simulink model "control_STMD_Ideal_Entrega_Final"  (R2021b)
settings: Solver=ode4  StartTime=0.0  StopTime=tend  FixedStep=ts  RelTol=1e-3  EnableMultiTasking=on
values from neighbouring files (symbols this model uses):
  ct = 2*mt*(2*pi*ft)*dampt    [script_control_STMD_Ideal_Entrega_Final.m]
  Kmax = 1*ct    [script_control_STMD_Ideal_Entrega_Final.m]
  Kmin = ct/2    [script_control_STMD_Ideal_Entrega_Final.m]
  kt = ((2*pi*ft)^2)*mt    [script_control_STMD_Ideal_Entrega_Final.m]
  mt = mu*m1    (= 60)    [script_control_STMD_Ideal_Entrega_Final.m]
  tend = 15    [script_control_STMD_Ideal_Entrega_Final.m]
  ts = 1/fs    (= 0.000666666666667)    [script_control_STMD_Ideal_Entrega_Final.m]
  u_active = 200    [script_control_STMD_Ideal_Entrega_Final.m]
undefined symbols (not defined in the file or in its folder): D_Gs, N_Gs
libraries: simulink x1
settings Model: Creator=user  LastModifiedBy=luismiguelmartinezgomez
settings SolverCC: AlgebraicLoopSolver=TrustRegion
settings DataIOCC: LimitDataPoints=on  SaveFormat=Array  SignalLoggingSaveFormat=ModelDataLogs  ReturnWorkspaceOutputs=off  SignalLoggingName=sigsOut
settings OptimizationCC: InitFltsAndDblsToZero=on  LifeSpan=inf
settings DebuggingCC: SaveWithParameterizedLinksMsg=none  UnderspecifiedInitializationDetection=Classic  MergeDetectMultiDrivingBlocksExec=none  SignalResolutionControl=TryResolveAllWithWarning  MultiTaskDSMMsg=warning  MultiTaskCondExecSysMsg=none  FcnCallInpInsideContextMsg=warning  SFUnexpectedBacktrackingDiag=warning  SFNoUnconditionalDefaultTransitionDiag=warning  SFMachineParentedDataDiag=warning  ArithmeticOperatorsInVariantConditions=warning
settings HardwareCC: ProdBitPerPointer=32  ProdBitPerSizeT=32  ProdBitPerPtrDiffT=32  ProdLargestAtomicFloat=None  ProdIntDivRoundTo=Undefined  ProdEndianess=Unspecified  ProdWordSize=32  ProdHWDeviceType=32-bit Generic  TargetBitPerLong=64  TargetBitPerPointer=64  TargetBitPerSizeT=64  TargetBitPerPtrDiffT=64  TargetLongLongMode=on  TargetIntDivRoundTo=Zero  TargetEndianess=LittleEndian  TargetWordSize=64  TargetHWDeviceType=MATLAB Host  ProdEqTarget=off
settings ModelReferenceCC: PropagateSignalLabelsOutOfModel=off
settings SFSimCC: SimUseLocalCustomCode=off  CustomCodeUndefinedFunction=UseInterfaceOnly
settings RTWCC: RTWUseLocalCustomCode=off
settings CodeAppCC: StateflowObjectComments=on
settings GRTTargetCC: TargetFcnLib=ansi_tfl_tmw.mat  TargetLangStandard=C89/C90 (ANSI)  CombineOutputUpdateFcns=off  GRTInterface=on
settings ConfigComp: CovMetricSettings=dw  CovSaveCumulativeToWorkspaceVar=on  CovSaveSingleToWorkspaceVar=on  CovExternalEMLEnable=off  CovSFcnEnable=off

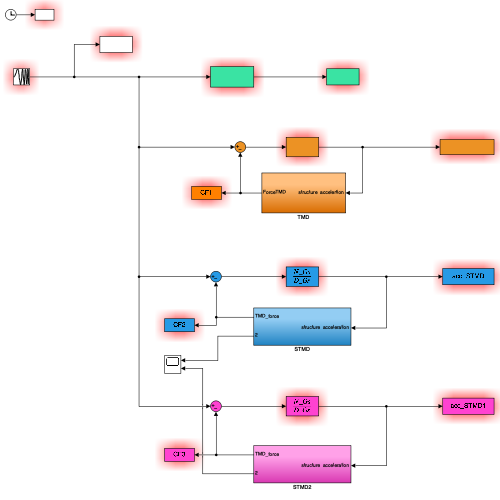
[thumbnail: Simulink's stored preview of the top-level diagram]
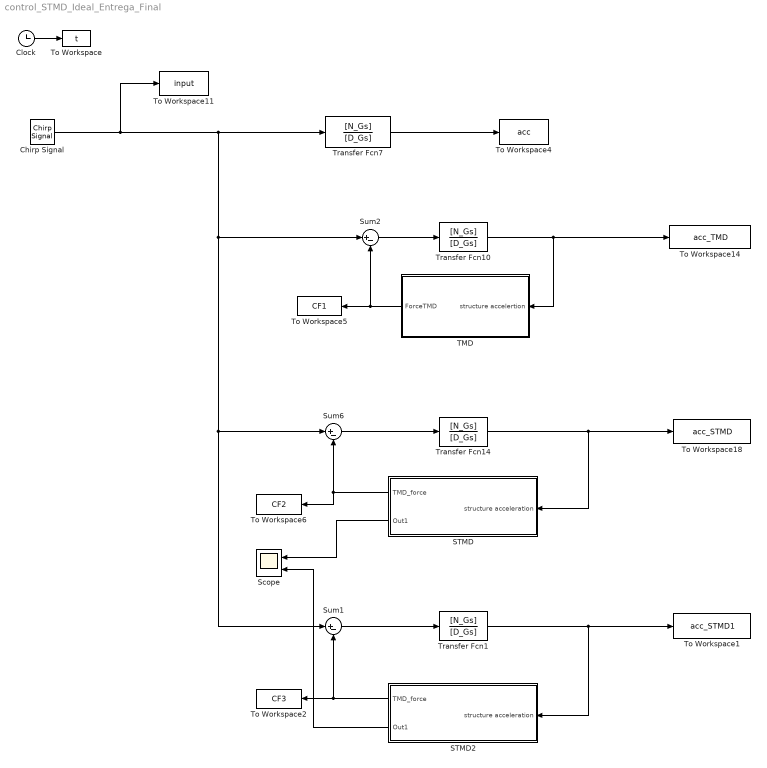
== system control_STMD_Ideal_Entrega_Final ==
  Chirp Signal : simulink/Sources/Chirp Signal  f1=fmin  T=tend  f2=fmax
  Clock : Clock
  STMD : Subsystem
  STMD2 : Subsystem
  Scope : Scope  NumInputPorts=2
  Sum1 : Sum  Inputs=|+-
  Sum2 : Sum  Inputs=|+-
  Sum6 : Sum  Inputs=|+-
  TMD : Subsystem
  To Workspace : ToWorkspace  VariableName=t  SampleTime=ts
  To Workspace1 : ToWorkspace  VariableName=acc_STMD1  SampleTime=ts
  To Workspace11 : ToWorkspace  VariableName=input  SampleTime=ts
  To Workspace14 : ToWorkspace  VariableName=acc_TMD  SampleTime=ts
  To Workspace18 : ToWorkspace  VariableName=acc_STMD  SampleTime=ts
  To Workspace2 : ToWorkspace  VariableName=CF3  SampleTime=ts
  To Workspace4 : ToWorkspace  VariableName=acc  SampleTime=ts
  To Workspace5 : ToWorkspace  VariableName=CF1  SampleTime=ts
  To Workspace6 : ToWorkspace  VariableName=CF2  SampleTime=ts
  Transfer Fcn{1,7,10,14} (4 alike) : TransferFcn  Numerator=[N_Gs]  Denominator=[D_Gs]
  wires:
  Clock/1 -> To Workspace/1
  Sum2/1 -> Transfer Fcn10/1
  TMD/1(ForceTMD) -> Sum2/2, To Workspace5/1
  Transfer Fcn7/1 -> To Workspace4/1
  Transfer Fcn10/1 -> TMD/1(structure accelertion), To Workspace14/1
  Sum6/1 -> Transfer Fcn14/1
  Transfer Fcn14/1 -> STMD/1(structure acceleration), To Workspace18/1
  STMD/1(TMD_force) -> To Workspace6/1, Sum6/2
  Chirp Signal/1 -> Sum2/1, Sum1/1, Sum6/1, Transfer Fcn7/1, To Workspace11/1
  STMD2/1(TMD_force) -> Sum1/2, To Workspace2/1
  Transfer Fcn1/1 -> STMD2/1(structure acceleration), To Workspace1/1
  Sum1/1 -> Transfer Fcn1/1
  STMD/2(Out1) -> Scope/1
  STMD2/2(Out1) -> Scope/2

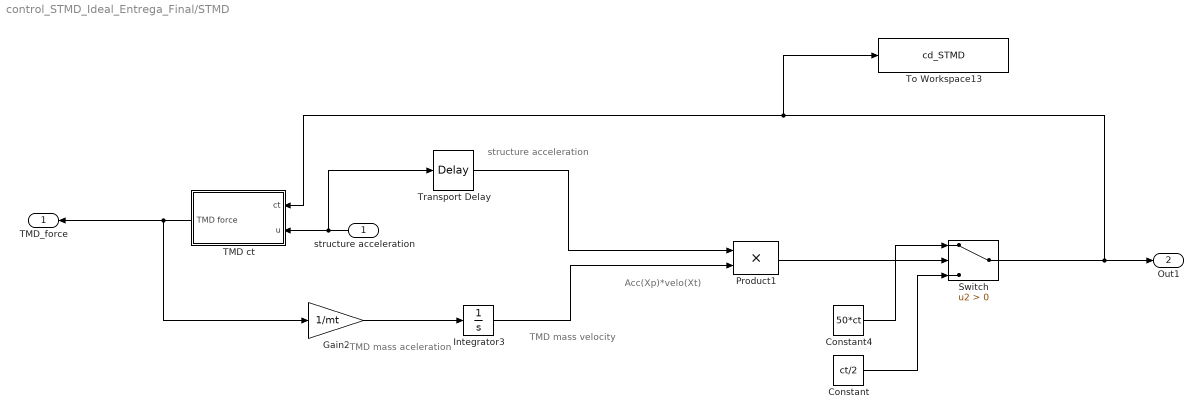
== system control_STMD_Ideal_Entrega_Final/STMD ==
  note: structure acceleration
  note: TMD mass
      | aceleration
  note: Acc(Xp)*velo(Xt)
  note: TMD mass
      | velocity
  structure acceleration : Inport
  Constant : Constant  Value=ct/2
  Constant4 : Constant  Value=50*ct
  Gain2 : Gain  Gain=1/mt
  Integrator3 : Integrator
  Product1 : Product  OutDataTypeStr=double  SaturateOnIntegerOverflow=on
  Switch : Switch  Criteria=u2 > Threshold
  TMD ct : Subsystem
  To Workspace13 : ToWorkspace  VariableName=cd_STMD  SampleTime=ts
  Transport Delay : TransportDelay  DelayTime=ts
  TMD_force : Outport  VectorParamsAs1DForOutWhenUnconnected=off
  Out1 : Outport  Port=2
  wires:
  TMD ct/1(TMD force) -> Gain2/1, TMD_force/1
  Integrator3/1 -> Product1/2
  Switch/1 -> Out1/1, To Workspace13/1, TMD ct/1(ct)
  structure acceleration/1 -> Transport Delay/1, TMD ct/2(u)
  Transport Delay/1 -> Product1/1
  Gain2/1 -> Integrator3/1
  Product1/1 -> Switch/2
  Constant4/1 -> Switch/1
  Constant/1 -> Switch/3

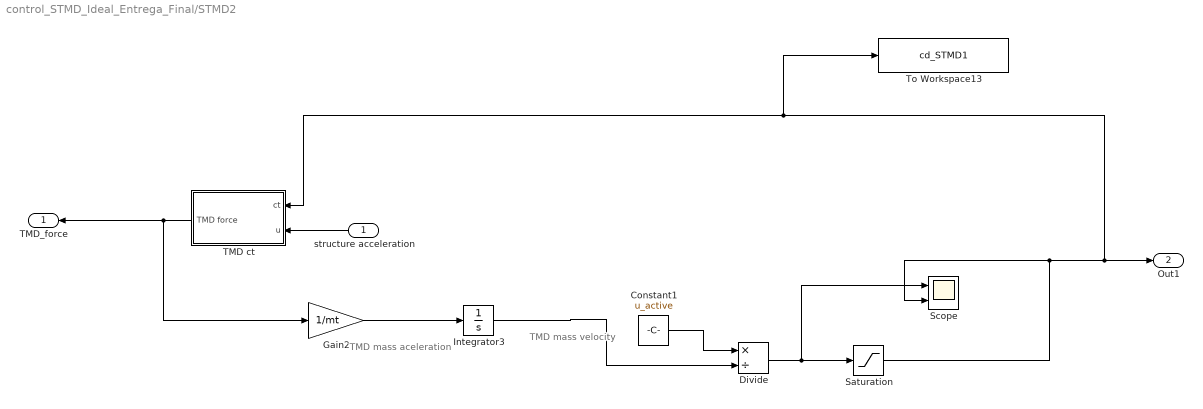
== system control_STMD_Ideal_Entrega_Final/STMD2 ==
  note: TMD mass
      | velocity
  note: TMD mass
      | aceleration
  structure acceleration : Inport
  Constant1 : Constant  Value=u_active
  Divide : Product  Inputs=*/
  Gain2 : Gain  Gain=1/mt
  Integrator3 : Integrator
  Saturation : Saturate  UpperLimit=Kmax  LowerLimit=Kmin
  Scope : Scope  NumInputPorts=2
  TMD ct : Subsystem
  To Workspace13 : ToWorkspace  VariableName=cd_STMD1  SampleTime=ts
  TMD_force : Outport  VectorParamsAs1DForOutWhenUnconnected=off
  Out1 : Outport  Port=2
  wires:
  Divide/1 -> Scope/1, Saturation/1
  Gain2/1 -> Integrator3/1
  structure acceleration/1 -> TMD ct/2(u)
  Integrator3/1 -> Divide/2
  TMD ct/1(TMD force) -> TMD_force/1, Gain2/1
  Saturation/1 -> Scope/2, TMD ct/1(ct), To Workspace13/1, Out1/1
  Constant1/1 -> Divide/1

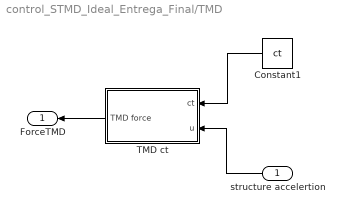
== system control_STMD_Ideal_Entrega_Final/TMD ==
  structure accelertion : Inport
  Constant1 : Constant  Value=ct
  TMD ct : Subsystem
  ForceTMD : Outport  VectorParamsAs1DForOutWhenUnconnected=off
  wires:
  TMD ct/1(TMD force) -> ForceTMD/1
  structure accelertion/1 -> TMD ct/2(u)
  Constant1/1 -> TMD ct/1(ct)

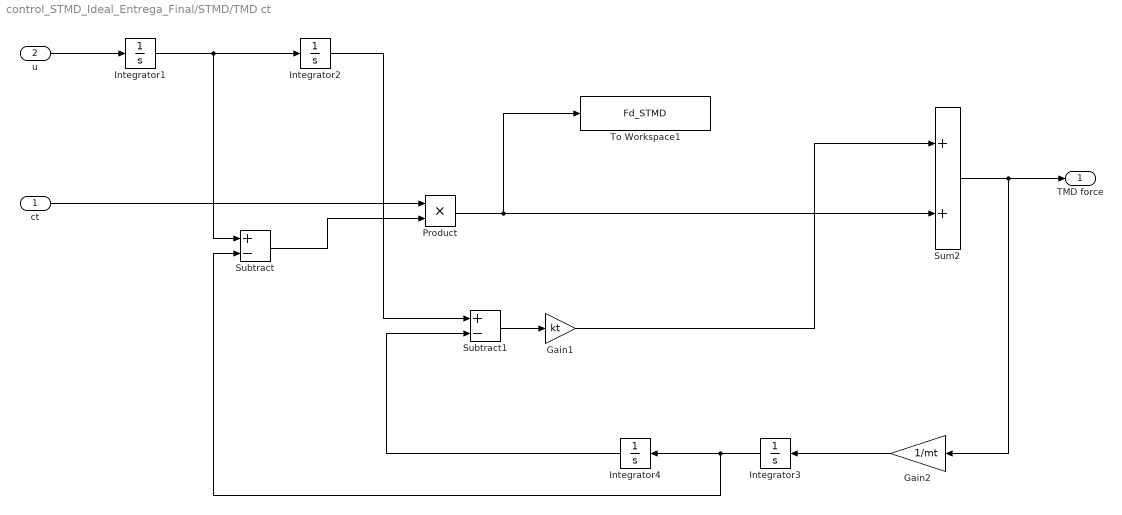
== system control_STMD_Ideal_Entrega_Final/STMD/TMD ct ==
  ct : Inport
  u : Inport  Port=2
  Gain1 : Gain  Gain=kt
  Gain2 : Gain  Gain=1/mt
  Integrator{1..4} (4 alike) : Integrator
  Product : Product
  Subtract : Sum  Inputs=+-
  Subtract1 : Sum  Inputs=+-
  Sum2 : Sum
  To Workspace1 : ToWorkspace  VariableName=Fd_STMD  SampleTime=ts
  TMD force : Outport  VectorParamsAs1DForOutWhenUnconnected=off
  wires:
  Integrator1/1 -> Subtract/1, Integrator2/1
  u/1 -> Integrator1/1
  Integrator3/1 -> Integrator4/1, Subtract/2
  Gain2/1 -> Integrator3/1
  Integrator4/1 -> Subtract1/2
  Integrator2/1 -> Subtract1/1
  Subtract1/1 -> Gain1/1
  Gain1/1 -> Sum2/1
  Sum2/1 -> Gain2/1, TMD force/1
  ct/1 -> Product/1
  Subtract/1 -> Product/2
  Product/1 -> Sum2/2, To Workspace1/1

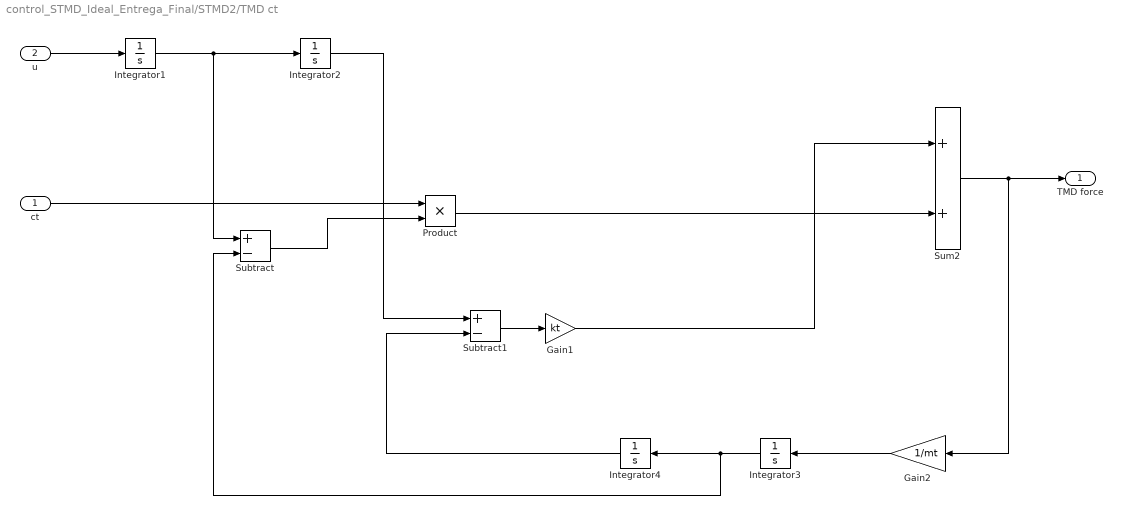
== system control_STMD_Ideal_Entrega_Final/STMD2/TMD ct ==
  ct : Inport
  u : Inport  Port=2
  Gain1 : Gain  Gain=kt
  Gain2 : Gain  Gain=1/mt
  Integrator{1..4} (4 alike) : Integrator
  Product : Product
  Subtract : Sum  Inputs=+-
  Subtract1 : Sum  Inputs=+-
  Sum2 : Sum
  TMD force : Outport  VectorParamsAs1DForOutWhenUnconnected=off
  wires:
  Product/1 -> Sum2/2
  Subtract/1 -> Product/2
  ct/1 -> Product/1
  Sum2/1 -> TMD force/1, Gain2/1
  Gain1/1 -> Sum2/1
  Subtract1/1 -> Gain1/1
  Integrator2/1 -> Subtract1/1
  Integrator4/1 -> Subtract1/2
  Gain2/1 -> Integrator3/1
  Integrator3/1 -> Subtract/2, Integrator4/1
  u/1 -> Integrator1/1
  Integrator1/1 -> Integrator2/1, Subtract/1

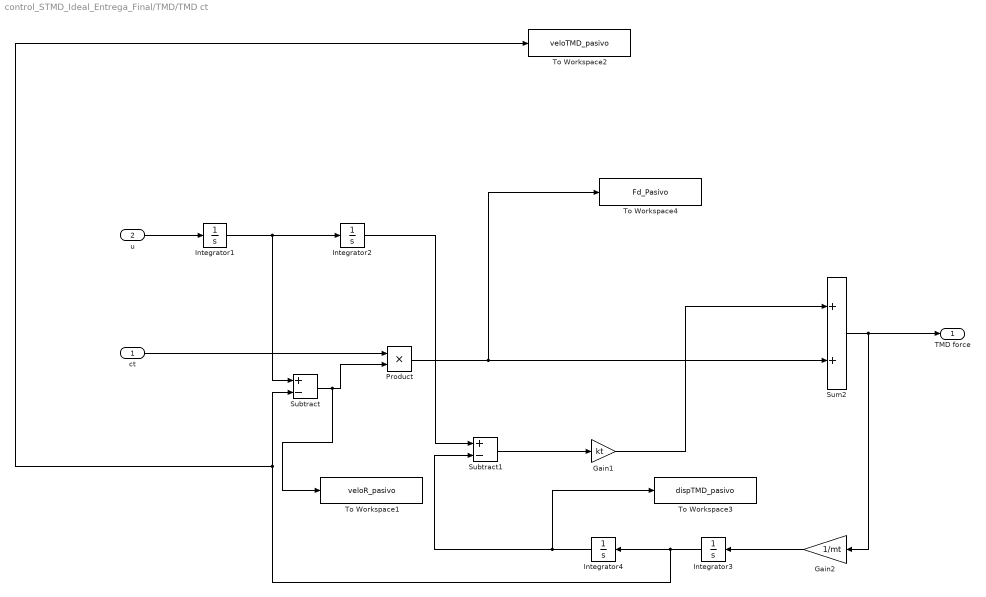
== system control_STMD_Ideal_Entrega_Final/TMD/TMD ct ==
  ct : Inport
  u : Inport  Port=2
  Gain1 : Gain  Gain=kt
  Gain2 : Gain  Gain=1/mt
  Integrator{1..4} (4 alike) : Integrator
  Product : Product
  Subtract : Sum  Inputs=+-
  Subtract1 : Sum  Inputs=+-
  Sum2 : Sum
  To Workspace1 : ToWorkspace  VariableName=veloR_pasivo  SampleTime=ts
  To Workspace2 : ToWorkspace  VariableName=veloTMD_pasivo  SampleTime=ts
  To Workspace3 : ToWorkspace  VariableName=dispTMD_pasivo  SampleTime=ts
  To Workspace4 : ToWorkspace  VariableName=Fd_Pasivo  SampleTime=ts
  TMD force : Outport  VectorParamsAs1DForOutWhenUnconnected=off
  wires:
  Integrator1/1 -> Subtract/1, Integrator2/1
  u/1 -> Integrator1/1
  ct/1 -> Product/1
  Integrator3/1 -> Integrator4/1, To Workspace2/1, Subtract/2
  Subtract/1 -> To Workspace1/1, Product/2
  Gain2/1 -> Integrator3/1
  Integrator4/1 -> To Workspace3/1, Subtract1/2
  Integrator2/1 -> Subtract1/1
  Subtract1/1 -> Gain1/1
  Gain1/1 -> Sum2/1
  Sum2/1 -> Gain2/1, TMD force/1
  Product/1 -> Sum2/2, To Workspace4/1
